simulink model "Ans8_Robo1_openloop"  (R2022b)
settings: Solver=VariableStepAuto  StartTime=0.0  StopTime=500  RelTol=1e-3
undefined symbols (not defined in the file or in its folder): sigbuilder_block
settings Model: Creator=SysIDEA_OSACE  LastModifiedBy=SysIDEA_OSACE

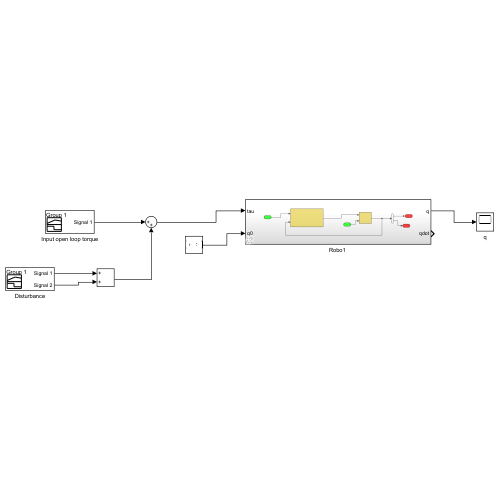
[thumbnail: Simulink's stored preview of the top-level diagram]
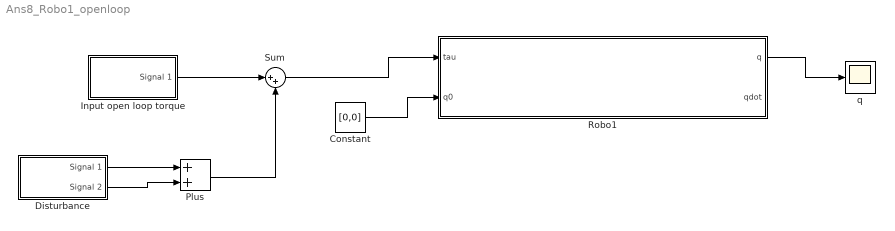
== system Ans8_Robo1_openloop ==
  Constant : Constant  Value=[0,0]
  Disturbance : Subsystem  Tag=STV Subsys  LoadFcn=sigbuilder_block('load',[721.5 235.5 550.5 399.75 ]);  StartFcn=sigbuilder_block('start');  StopFcn=sigbuilder_block('stop');  ClipboardFcn=sigbuilder_block('clipboard');  mask(Sigbuilder block){tuvar=[0:10]}
      mask help: Simulink:masks:SigbuilderBlock_MD
      mask init:
      | if ~strcmp(get_param(bdroot(gcbh),'SimulationStatus'),'stopped') tuvar = sigbuilder_block('maskInit'); end
      settings: CopyFcn=sigbuilder_block('copy');  DeleteFcn=sigbuilder_block('delete');  ModelCloseFcn=sigbuilder_block('modelClose');  PreSaveFcn=sigbuilder_block('preSave');  PauseFcn=sigbuilder_block('pause');  ContinueFcn=sigbuilder_block('continue');  NameChangeFcn=sigbuilder_block('namechange');  OpenFcn=sigbuilder_block('open',[437.6 199.2 550.4 400 ]);  CloseFcn=sigbuilder_block('close');
      mask Display: plot(0, 0, 100, 100,[2, 2, 32, 32, 2], [68, 8, 8, 68, 68],[32, 2], [38, 38], [32, 19, 2],[53, 60, 44], [32, 17, 17, 2],[16, 16, 31, 31]);txt = getActiveGroup(gcbh);text(2, 100, txt,'verticalAlignment', 'top');
  Input open loop torque : Subsystem  Tag=STV Subsys  LoadFcn=sigbuilder_block('load');  StartFcn=sigbuilder_block('start');  StopFcn=sigbuilder_block('stop');  ClipboardFcn=sigbuilder_block('clipboard');  mask(Sigbuilder block){tuvar=[0:10]}
      mask help: Simulink:masks:SigbuilderBlock_MD
      mask init:
      | if ~strcmp(get_param(bdroot(gcbh),'SimulationStatus'),'stopped') tuvar = sigbuilder_block('maskInit'); end
      settings: CopyFcn=sigbuilder_block('copy');  DeleteFcn=sigbuilder_block('delete');  ModelCloseFcn=sigbuilder_block('modelClose');  PreSaveFcn=sigbuilder_block('preSave');  PauseFcn=sigbuilder_block('pause');  ContinueFcn=sigbuilder_block('continue');  NameChangeFcn=sigbuilder_block('namechange');  OpenFcn=sigbuilder_block('open',[437.6 199.2 550.4 400 ]);  CloseFcn=sigbuilder_block('close');
      mask Display: plot(0, 0, 100, 100,[2, 2, 32, 32, 2], [68, 8, 8, 68, 68],[32, 2], [38, 38], [32, 19, 2],[53, 60, 44], [32, 17, 17, 2],[16, 16, 31, 31]);txt = getActiveGroup(gcbh);text(2, 100, txt,'verticalAlignment', 'top');
  Plus : Sum
  "Robo1 " : Subsystem  AncestorBlock=mssSimulink/Marine craft models/Remus 100 AUV (remus100.m)
      settings: LibrarySourceBlock=mssSimulink/Marine craft models/Remus 100 AUV (remus100.m)
  Sum : Sum  Inputs=|++
  q : Scope
  wires:
  Constant/1 -> "Robo1 "/2(q0)
  Sum/1 -> "Robo1 "/1(tau)
  "Robo1 "/1(q) -> q/1
  Disturbance/1(Signal 1) -> Plus/1
  Disturbance/2(Signal 2) -> Plus/2
  Plus/1 -> Sum/2
  Input open loop torque/1(Signal 1) -> Sum/1

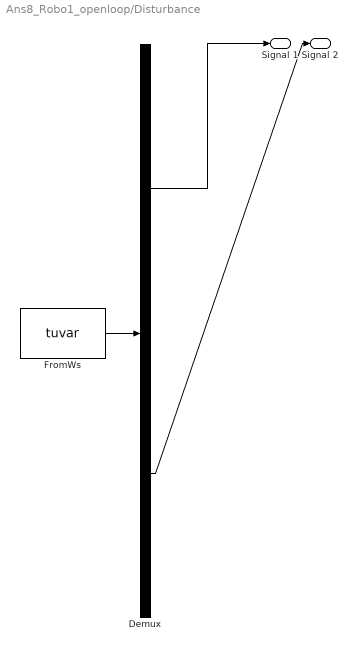
== system Ans8_Robo1_openloop/Disturbance ==
  Demux : Demux  Tag=STV Demux  Outputs=2
      settings: DisplayOption=none
  FromWs : FromWorkspace  Tag=STV FromWs  VariableName=tuvar
      SigBuilderData=|
      | common.afterFinalStr = 'Extrapolate'
      | common.sampleTime = 0
      | dataSet.timeRange = [0 10]
      | dataSet.name = 'Group 1'
      | sbobj.Groups.Name = 'Group 1'
      | sbobj.Groups.Signals(1).Name = 'Signal 1'
      | sbobj.Groups.Signals(1).XData = [0 4 4 6 6 10]
      | sbobj.Groups.Signals(1).YData = [0 0 0.995 0.995 0 0]
      | sbobj.Groups.Signals(2).Name = 'Signal 2'
      | sbobj.Groups.Signals(2).XData = [0 0.0166666666667 0.0333333333333 0.05 0.0666666666667 0.0833333333333 0.1 0.116666666667 0.133333333333 0.15 0.166666666667 0.183333333333 ... (601 elements, 1x601)]
      | sbobj.Groups.Signals(2).YData = [-0.888032082329 0.100092833139 -0.544528929991 0.303520794649 -0.600326562134 0.489965321174 0.739363123604 1.71188778298 -0.194123535758 -2.13835526944 -0.839588747337 1.354594328 ... (601 elements, 1x601)]
  Signal 1 : Outport  Tag=STV Outport
  Signal 2 : Outport  Tag=STV Outport  Port=2
  wires:
  Demux/1 -> Signal 1/1
  FromWs/1 -> Demux/1
  Demux/2 -> Signal 2/1

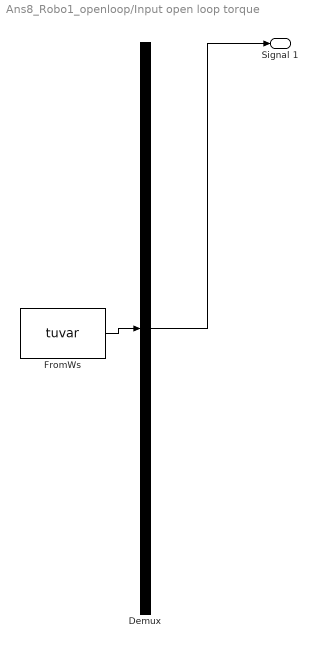
== system Ans8_Robo1_openloop/Input open loop torque ==
  Demux : Demux  Tag=STV Demux  Outputs=1
      settings: DisplayOption=none
  FromWs : FromWorkspace  Tag=STV FromWs  VariableName=tuvar
      SigBuilderData=|
      | common.afterFinalStr = 'Extrapolate'
      | common.sampleTime = 0
      | dataSet.timeRange = [0 10]
      | dataSet.name = 'Group 1'
      | sbobj.Groups.Name = 'Group 1'
      | sbobj.Groups.Signals.Name = 'Signal 1'
      | sbobj.Groups.Signals.XData = [0 5 5 10]
      | sbobj.Groups.Signals.YData = [-0.005 -0.005 1 1]
  Signal 1 : Outport  Tag=STV Outport
  wires:
  FromWs/1 -> Demux/1
  Demux/1 -> Signal 1/1

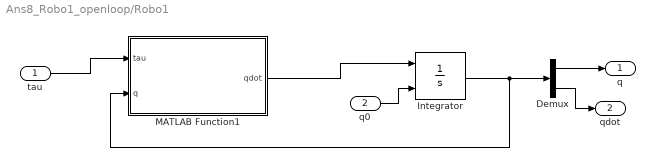
== system Ans8_Robo1_openloop/Robo1  ==
  tau : Inport
  q0 : Inport  Port=2
  Demux : Demux  Outputs=2
  Integrator : Integrator  InitialConditionSource=external  InitialCondition=[1 1]  UpperSaturationLimit=10  LowerSaturationLimit=-10
  MATLAB Function1 : MATLAB Function  TreatAsAtomicUnit=on
  q : Outport
  qdot : Outport  Port=2
  wires:
  MATLAB Function1/1(qdot) -> Integrator/1
  q0/1 -> Integrator/2
  Integrator/1 -> Demux/1, MATLAB Function1/2(q)
  tau/1 -> MATLAB Function1/1(tau)
  Demux/1 -> q/1
  Demux/2 -> qdot/1

== matlab function Ans8_Robo1_openloop/Robo1 /MATLAB Function1 ==
  data: tau input; qdot output; q input
function qdot  = fcn(tau,q)

  [qdot] = Robo1(tau,q);

end
